simulink model "controller_observer"  (R2015a)
settings: Solver=ode45  SolverMode=SingleTasking  StartTime=0.0  StopTime=10.0  RelTol=1e-3
values from neighbouring files (symbols this model uses):
  Ac = A-B*K-L*C    [cee_SCRIPT.m]
  Bc = L    [cee_SCRIPT.m]
  C = [1 0 0 0 0;0 0 1 0 0]    [cee_SCRIPT.m]
  Cc = -K    [cee_SCRIPT.m]
  D = [0;0]    [cee_SCRIPT.m]
  Dc = [0 0]    [cee_SCRIPT.m]
  x0 = [0 0 0 0 0]    [cee_SCRIPT.m]
  x0c = deg2rad(x0c_graus)'    [cee_SCRIPT.m]
undefined symbols (not defined in the file or in its folder): A, B
settings Model: CovMetricSettings=dwe  CovHtmlReporting=off  covSaveCumulativeToWorkspaceVar=off  CovSaveSingleToWorkspaceVar=off  CovExternalEMLEnable=on  Creator=jmgri  LastModifiedBy=jmgri
settings DataIOCC: LimitDataPoints=off  SaveFormat=Dataset
settings DebuggingCC: SFUnexpectedBacktrackingDiag=error  SFNoUnconditionalDefaultTransitionDiag=error
settings HardwareCC: ProdBitPerPointer=64  ProdLargestAtomicFloat=Float  ProdIntDivRoundTo=Zero  ProdEndianess=LittleEndian  ProdHWDeviceType=Specified
settings ModelReferenceCC: PropagateSignalLabelsOutOfModel=on
settings GRTTargetCC: TargetLangStandard=C99 (ISO)  GeneratePreprocessorConditionals=Use local settings

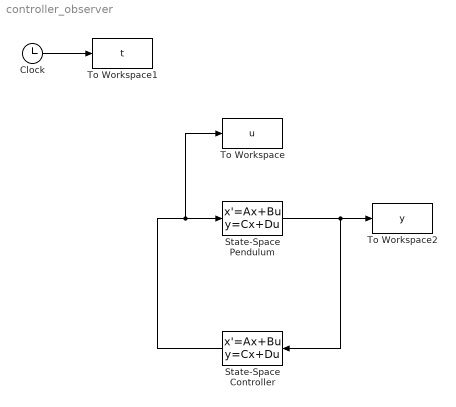
== system controller_observer ==
  Clock : Clock
  State-Space Controller : StateSpace  A=Ac  B=Bc  C=Cc  D=Dc  X0=x0c
  State-Space Pendulum : StateSpace  A=A  B=B  C=C  D=D  X0=x0
  To Workspace : ToWorkspace  VariableName=u  SampleTime=-1
  To Workspace1 : ToWorkspace  VariableName=t  SampleTime=-1
  To Workspace2 : ToWorkspace  VariableName=y  SampleTime=-1
  wires:
  Clock/1 -> To Workspace1/1
  State-Space Pendulum/1 -> State-Space Controller/1, To Workspace2/1
  State-Space Controller/1 -> To Workspace/1, State-Space Pendulum/1
